simulink model "Execution_gyro_2_corrige"  (R2013a)
settings: Solver=FixedStepDiscrete  StartTime=0.0  StopTime=inf  RelTol=1e-3
libraries: arduino_io_lib x3
settings Model: Creator=Francois  LastModifiedBy=Propriétaire
settings DataIOCC: SignalLoggingSaveFormat=ModelDataLogs
settings OptimizationCC: ExpressionDepthLimit=2147483647
settings DebuggingCC: FcnCallInpInsideContextMsg=EnableAllAsWarning

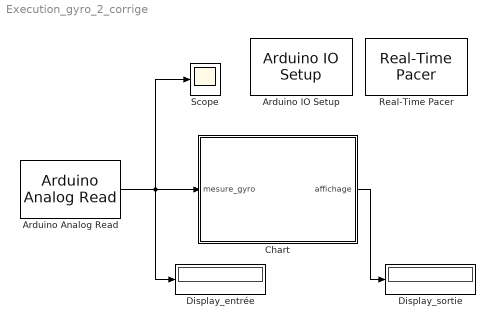
== system Execution_gyro_2_corrige ==
  Arduino Analog Read : arduino_io_lib/Arduino Analog Read  arduinoVar=Temporary arduino variable: Arduino1  arduinoPin=0  T=0.2
  Arduino IO Setup : arduino_io_lib/Arduino IO Setup  Priority=3  arduinoVar=Temporary arduino variable: Arduino1  workspaceVarName=a  comPort=COM49
  Chart : Stateflow chart  TreatAsAtomicUnit=on
  Display_entrée : Display
  Display_sortie : Display
  Real-Time Pacer : arduino_io_lib/Real-Time Pacer  simTimePerRealTime=1
  Scope : Scope
      settings: TimeRange=10  YMin=410  YMax=620
  wires:
  Arduino Analog Read/1 -> Chart/1(mesure_gyro), Display_entrée/1, Scope/1
  Chart/1(affichage) -> Display_sortie/1

== stateflow chart Execution_gyro_2_corrige/Chart ==
  state init_compteur
    entry : n = 0 ;
    affichage = n
  state memorise_1
    entry : memo_1 = mesure_gyro
  state memorise_2
    entry : memo_2 = mesure_gyro
  state calcule_ecart
    entry : ecart = memo_2 - memo_1;
    n = n+1;
    affichage = n
  state init_moyennage
    entry : compte =0;
    moyenne = 0; total = 0
  state memorise_3
    entry : memo_3 = mesure_gyro;
    compte = compte + 1
  state calcule_moyenne
    entry : total = total + memo_3;
    moyenne = total / compte;
    affichage = total
  state affiche_moyenne
    entry : affichage = moyenne
  (default) -> init_compteur
  calcule_ecart -> init_compteur [order 1] : [ecart >= 5]
  init_compteur -> memorise_1 : after(3,sec)
  (junction 121) -> memorise_1 [order 1] : [n<10]
  memorise_1 -> memorise_2 : after(0.1,sec)
  memorise_2 -> calcule_ecart
  calcule_ecart -> (junction 121) [order 2] : [ecart < 5]
  (junction 121) -> init_moyennage [order 2] : [n==10]
  init_moyennage -> memorise_3
  calcule_moyenne -> memorise_3 [order 1] : [compte < 50]
  memorise_3 -> calcule_moyenne : after(0.1,sec)
  calcule_moyenne -> affiche_moyenne [order 2] : [compte == 50]
  data: mesure_gyro input; affichage output double; ecart local double; memo_1 local double; memo_2 local double; memo_3 local double; moyenne local double; n local double; compte local double; total local double
